simulink model "IntegrationTestSim"  (R2018b)
settings: Solver=ode45  StartTime=0.0  StopTime=600  RelTol=1e-3  EnableMultiTasking=on
values from neighbouring files (symbols this model uses):
  enableHorzMan = 1    [IntegrationTestClass.m]
  enableVertMan = 0    [IntegrationTestClass.m]
  ignorePrevAlert = 1    [IntegrationTestClass.m]
  sim_sampleTime = 0.1    [IntegrationTestClass.m]
  uasSensorSelected = 1    [IntegrationTestClass.m]
  uasSurveillance_sampleTime = 0.1    [IntegrationTestClass.m]
undefined symbols (not defined in the file or in its folder): ac1dyn_alt0_ft, ac1dyn_lat0_rad, ac1dyn_lon0_rad, daa_turnRate_dps, daa_vertRate_fpm, dh_flag, dh_ftps, dpsi_flag, dpsi_radps, uasPilot_altitudeK, uasPilot_altitudeOffset, uasPilot_altitudeTheta, uasPilot_coordDelayK, uasPilot_coordDelayMin, uasPilot_coordDelayTheta, uasPilot_desiredTurnRate_dps, uasPilot_desiredVertRate_ftpm, uasPilot_deterministicMode, uasPilot_dt_s, uasPilot_executionDelayMin, uasPilot_executionDelayMu, uasPilot_initialDelayMin, uasPilot_initialDelayMu, uasPilot_maxRelativeHdg, uasPilot_meanUpdateTimes, uasPilot_mentalFilter_climbThresh_fps, uasPilot_mentalFilter_numSamp, uasPilot_mentalFilter_turnThresh_rad, uasPilot_minUpdateTimes, uasPilot_operatorEnabled, uasPilot_probDescend, uasPilot_probFollowMinDev, uasPilot_probLeftTurn, uasPilot_probTurn, uasPilot_reducedClimbAlt_ft, uasPilot_reducedTurnAngle_deg, uasPilot_seedChoose, uasPilot_seedCoordDelay, uasPilot_seedExecutionDelay, uasPilot_seedInitialDelay, uasPilot_seedTurn, uasPilot_seedUpdate, uasPilot_seedVertical, uasPilot_triggerLevel, uasPilot_turnK, uasPilot_turnOffset, uasPilot_turnTheta
libraries: simulink x4, BasicAircraftDynamicsBlock x3, NominalTrajectory x2, FlattenAircraftEstimateBus x2, PerfectSurveillanceBlock x2, sph2cart x2, DaidalusV201Block x1, HysteresisFilterBlock x1, MofNFilterBlock x1, CommonMetricsBlock x1, SLoWCBlock x1, WellClearMetricsBlock x1
(part 3 of 3)

== system IntegrationTestSim/Surveillance Source/Subsystem/Simple Tracked Surveillance ==
  Intruder Aircraft State : Inport
  Clock : Inport  Port=2
  Intruder Aircraft State Rate : Inport  Port=3
  Rate Transition : RateTransition  OutPortSampleTime=uasLogic_sampleTime
  Rate Transition1 : RateTransition  OutPortSampleTime=uasLogic_sampleTime
  Rate Transition2 : RateTransition  OutPortSampleTime=uasLogic_sampleTime
  Simple Tracked Surveillance : SimpleTrackedSurveillanceBlock/Simple Tracked Surveillance  horizontal_position_jitter_stddev_ft=ac1_ac2_horizontal_position_jitter_stddev_ft  vertical_position_jitter_stddev_ft=ac1_ac2_vertical_position_jitter_stddev_ft  horizontal_velocity_jitter_stddev_fps=ac1_ac2_horizontal_velocity_jitter_stddev_fps  vertical_velocity_jitter_stddev_fps=ac1_ac2_vertical_velocity_jitter_stddev_fps  nVar_ft2=ac1_ac2_nVar_ft2  eVar_ft2=ac1_ac2_eVar_ft2  hVar_ft2=ac1_ac2_hVar_ft2  dnVar_ft2ps2=ac1_ac2_dnVar_ft2ps2  deVar_ft2ps2=ac1_ac2_deVar_ft2ps2  dhVar_ft2ps2=ac1_ac2_dhVar_ft2ps2  seed1=ac1_ac2_seed1  seed2=ac1_ac2_seed2  seed3=ac1_ac2_seed3  seed4=ac1_ac2_seed4  seed5=ac1_ac2_seed5  seed6=ac1_ac2_seed6  east_position_error_ft=ac1_ac2_east_position_error_ft  north_position_error_ft=ac1_ac2_north_position_error_ft  vertical_position_error_ft=ac1_ac2_vertical_position_error_ft  east_velocity_error_fps=ac1_ac2_east_velocity_error_fps  north_velocity_error_fps=ac1_ac2_north_velocity_error_fps  vertical_velocity_error_fps=ac1_ac2_vertical_velocity_error_fps  lat0_rad=ac1dyn_lat0_rad  lon0_rad=ac1dyn_lon0_rad  alt0_ft=ac1dyn_alt0_ft
  Terminator : Terminator
  Intruder AircraftEstimate : Outport
  wires:
  Intruder Aircraft State/1 -> Rate Transition/1
  Intruder Aircraft State Rate/1 -> Rate Transition2/1
  Clock/1 -> Rate Transition1/1
  Simple Tracked Surveillance/2 -> Terminator/1
  Rate Transition/1 -> Simple Tracked Surveillance/1
  Rate Transition1/1 -> Simple Tracked Surveillance/2
  Rate Transition2/1 -> Simple Tracked Surveillance/3
  Simple Tracked Surveillance/1 -> Intruder AircraftEstimate/1

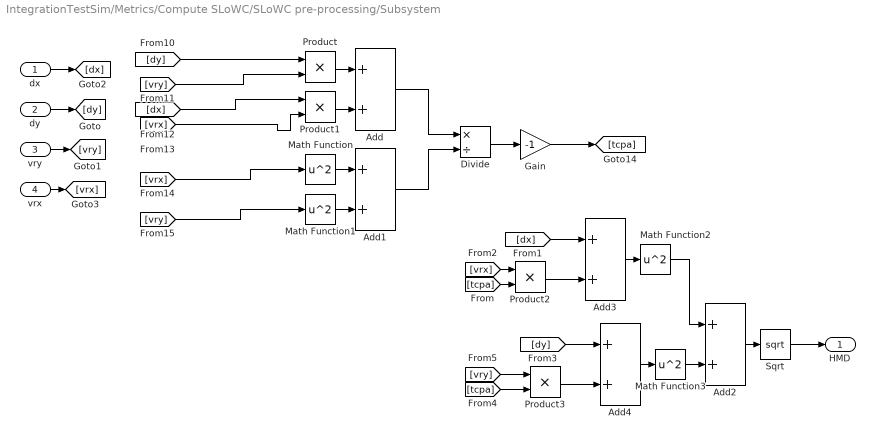
== system IntegrationTestSim/Metrics/Compute SLoWC/SLoWC pre-processing/Subsystem ==
  "dx " : Inport
  dy : Inport  Port=2
  vry : Inport  Port=3
  vrx : Inport  Port=4
  Add{,1..4} (5 alike) : Sum
  Divide : Product  Inputs=*/
  Gain : Gain  Gain=-1
  Math Function{,1..3} (4 alike) : Math  Operator=square  SaturateOnIntegerOverflow=on
  Product{,1..3} (4 alike) : Product
  Sqrt : Sqrt  SaturateOnIntegerOverflow=on
  HMD : Outport
  wires:
  Math Function1/1 -> Add1/2
  Gain/1 -> [tcpa]
  Add/1 -> Divide/1
  Math Function/1 -> Add1/1
  Product1/1 -> Add/2
  Product/1 -> Add/1
  [vrx] -> Math Function/1
  [vrx] -> Product1/2
  [dx] -> Product1/1
  Divide/1 -> Gain/1
  Add1/1 -> Divide/2
  [vry] -> Product/2
  [dy] -> Product/1
  [vry] -> Math Function1/1
  Sqrt/1 -> HMD/1
  Add2/1 -> Sqrt/1
  Math Function2/1 -> Add2/1
  Add3/1 -> Math Function2/1
  [dx] -> Add3/1
  [vrx] -> Product2/1
  Product2/1 -> Add3/2
  [tcpa] -> Product2/2
  Add4/1 -> Math Function3/1
  Math Function3/1 -> Add2/2
  Product3/1 -> Add4/2
  [dy] -> Add4/1
  [tcpa] -> Product3/2
  [vry] -> Product3/1
  "dx "/1 -> [dx]
  vrx/1 -> [vrx]
  vry/1 -> [vry]
  dy/1 -> [dy]

== system IntegrationTestSim/Metrics/Compute SLoWC/SLoWC pre-processing/Subsystem1 ==
  "int_n " : Inport
  own_n : Inport  Port=2
  int_e : Inport  Port=3
  own_e : Inport  Port=4
  Add1 : Sum
  Math Function : Math  Operator=square  SaturateOnIntegerOverflow=on
  Math Function1 : Math  Operator=square  SaturateOnIntegerOverflow=on
  Sqrt : Sqrt  SaturateOnIntegerOverflow=on
  Subtract5 : Sum  Inputs=+-
  Subtract6 : Sum  Inputs=+-
  Out1 : Outport
  wires:
  Math Function/1 -> Add1/1
  Add1/1 -> Sqrt/1
  Math Function1/1 -> Add1/2
  Subtract5/1 -> Math Function/1
  Sqrt/1 -> Out1/1
  Subtract6/1 -> Math Function1/1
  int_e/1 -> Subtract6/1
  own_n/1 -> Subtract5/2
  "int_n "/1 -> Subtract5/1
  own_e/1 -> Subtract6/2

== system IntegrationTestSim/Pilot/Format Maneuver As AircraftCommand/Horizontal Maneuver/Set Desired Turn Rate ==
  Cmd In : Inport
  Maneuver Magnitude : Inport  Port=2
  Own State : Inport  Port=3
  Bus Assignment1 : BusAssignment  AssignedSignals=dpsi_flag,dpsi_radps
  Constant : Constant  OutDataTypeStr=boolean
  Desired Heading to Turn Rate : Subsystem
  Cmd Out : Outport
  wires:
  Own State/1 -> Desired Heading to Turn Rate/2(Own State)
  Bus Assignment1/1 -> Cmd Out/1
  Cmd In/1 -> Bus Assignment1/1
  Constant/1 -> Bus Assignment1/2
  Maneuver Magnitude/1 -> Desired Heading to Turn Rate/1(Heading Cmd)
  Desired Heading to Turn Rate/1(Turn Rate) -> Bus Assignment1/3

== system IntegrationTestSim/Pilot/Format Maneuver As AircraftCommand/Vertical Maneuver/Set Desired Vertical Rate ==
  Cmd In : Inport
  Own State : Inport  Port=2
  Maneuver : Inport  Port=3
  dh_ftps : Inport  Port=4
  Bus Assignment : BusAssignment  AssignedSignals=dh_flag,dh_ftps
  Constant : Constant  OutDataTypeStr=boolean
  Constant1 : Constant  Value=enableVertMan
  Desired Altitude to Vertical Rate : Subsystem
  Multiport Switch : MultiPortSwitch  DataPortOrder=Specify indices  DataPortIndices={1 0}
  Scope : Scope
  Cmd Out : Outport
  wires:
  Bus Assignment/1 -> Cmd Out/1
  Own State/1 -> Desired Altitude to Vertical Rate/2(Own State)
  Cmd In/1 -> Bus Assignment/1
  Constant/1 -> Bus Assignment/2
  Maneuver/1 -> Desired Altitude to Vertical Rate/1(Altitude Cmd)
  dh_ftps/1 -> Multiport Switch/3
  Constant1/1 -> Multiport Switch/1
  Desired Altitude to Vertical Rate/1(Vert Rt) -> Scope/1, Multiport Switch/2
  Multiport Switch/1 -> Bus Assignment/3

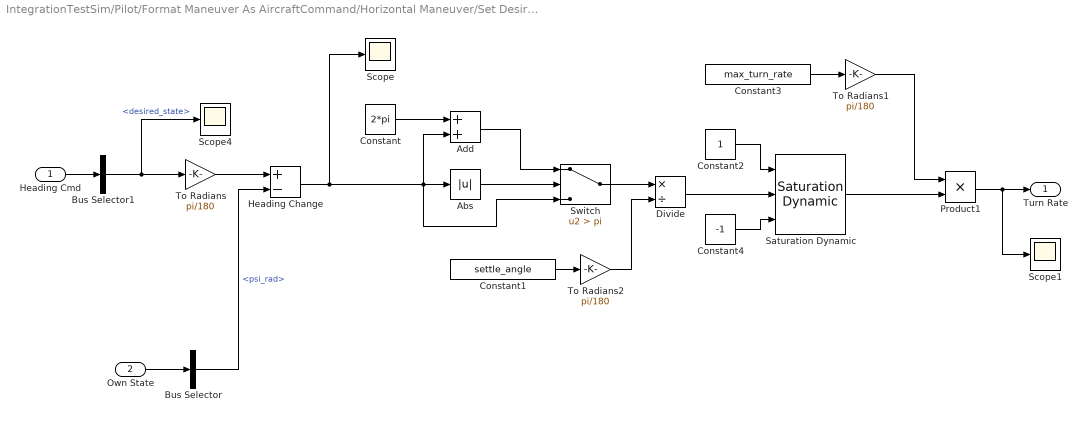
== system IntegrationTestSim/Pilot/Format Maneuver As AircraftCommand/Horizontal Maneuver/Set Desired Turn Rate/Desired Heading to Turn Rate ==
  Heading Cmd : Inport
  Own State : Inport  Port=2
  Abs : Abs
  Add : Sum
  Bus Selector : BusSelector  OutputSignals=psi_rad
  Bus Selector1 : BusSelector  OutputSignals=desired_state
  Constant : Constant  Value=2*pi
  Constant1 : Constant  Value=settle_angle
  Constant2 : Constant
  Constant3 : Constant  Value=max_turn_rate
  Constant4 : Constant  Value=-1
  Divide : Product  Inputs=*/
  Heading Change : Sum  Inputs=+-
  Product1 : Product  RndMeth=Zero
  Saturation Dynamic : simulink/Discontinuities/Saturation Dynamic  OutMin=[]  OutMax=[]  OutDataTypeStr=Inherit: Same as second input  OutDataType=fixdt(1, 16)  OutScaling=2^-10  DoSatur=off
  Scope : Scope
  Scope1 : Scope
  Scope4 : Scope
  Switch : Switch  Criteria=u2 > Threshold  Threshold=pi
  To Radians : Gain  Gain=pi/180
  To Radians1 : Gain  Gain=pi/180
  To Radians2 : Gain  Gain=pi/180
  Turn Rate : Outport
  wires:
  Constant/1 -> Add/1
  Switch/1 -> Divide/1
  Constant4/1 -> Saturation Dynamic/3
  Divide/1 -> Saturation Dynamic/2
  Abs/1 -> Switch/2
  Heading Change/1 -> Scope/1, Switch/3, Abs/1, Add/2
  Add/1 -> Switch/1
  Own State/1 -> Bus Selector/1
  Bus Selector/1 -> Heading Change/2  "<psi_rad>"
  To Radians/1 -> Heading Change/1
  Constant2/1 -> Saturation Dynamic/1
  Saturation Dynamic/1 -> Product1/2
  Constant1/1 -> To Radians2/1
  Product1/1 -> Scope1/1, Turn Rate/1
  Constant3/1 -> To Radians1/1
  To Radians1/1 -> Product1/1
  To Radians2/1 -> Divide/2
  Bus Selector1/1 -> To Radians/1, Scope4/1  "<desired_state>"
  Heading Cmd/1 -> Bus Selector1/1

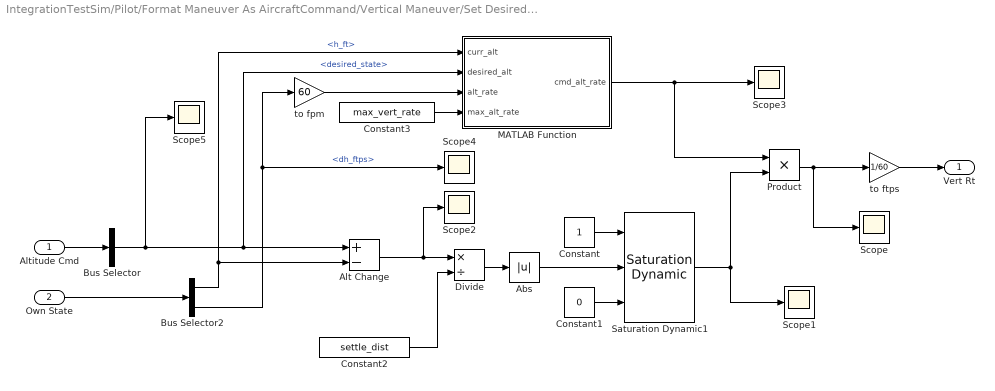
== system IntegrationTestSim/Pilot/Format Maneuver As AircraftCommand/Vertical Maneuver/Set Desired Vertical Rate/Desired Altitude to Vertical Rate ==
  Altitude Cmd : Inport
  Own State : Inport  Port=2
  Abs : Abs
  Alt Change : Sum  Inputs=+-
  Bus Selector : BusSelector  OutputSignals=desired_state
  Bus Selector2 : BusSelector  OutputSignals=h_ft,dh_ftps
  Constant : Constant
  Constant1 : Constant  Value=0
  Constant2 : Constant  Value=settle_dist
  Constant3 : Constant  Value=max_vert_rate
  Divide : Product  Inputs=*/
  MATLAB Function : MATLAB Function  TreatAsAtomicUnit=on
  Product : Product  RndMeth=Zero
  Saturation Dynamic1 : simulink/Discontinuities/Saturation Dynamic  OutMin=[]  OutMax=[]  OutDataTypeStr=Inherit: Same as second input  OutDataType=fixdt(1, 16)  OutScaling=2^-10  DoSatur=off
  Scope{,1..5} (6 alike) : Scope
  to fpm : Gain  Gain=60
  to ftps : Gain  Gain=1/60
  Vert Rt : Outport
  wires:
  Constant2/1 -> Divide/2
  Alt Change/1 -> Divide/1, Scope2/1
  Product/1 -> to ftps/1, Scope/1
  Own State/1 -> Bus Selector2/1
  Altitude Cmd/1 -> Bus Selector/1
  Bus Selector2/1 -> MATLAB Function/1(curr_alt), Alt Change/2  "<h_ft>"
  Divide/1 -> Abs/1
  Constant/1 -> Saturation Dynamic1/1
  Constant1/1 -> Saturation Dynamic1/3
  Saturation Dynamic1/1 -> Scope1/1, Product/2
  Abs/1 -> Saturation Dynamic1/2
  to ftps/1 -> Vert Rt/1
  Bus Selector/1 -> Scope5/1, MATLAB Function/2(desired_alt), Alt Change/1  "<desired_state>"
  Constant3/1 -> MATLAB Function/4(max_alt_rate)
  Bus Selector2/2 -> Scope4/1, to fpm/1  "<dh_ftps>"
  MATLAB Function/1(cmd_alt_rate) -> Scope3/1, Product/1
  to fpm/1 -> MATLAB Function/3(alt_rate)

== matlab function IntegrationTestSim/Surveillance Source/Subsystem/SC-228 Active Surveillance (Tracked)/MATLAB Function ==
  data: lat0 input double; lon0 input double; h0 input double; n_ft input double; e_ft input double size=1; u_ft input double; vn_ftps input double; ve_ftps input double; vh_ftps input double; lat_rad output double; lon_rad output double; dlat_radps output double; dlon_radps output double; alt_ft output double; dalt_ftps output double
function [lat_rad,lon_rad,dlat_radps,dlon_radps,alt_ft,dalt_ftps] = convertToLLA(lat0,lon0,h0,n_ft,e_ft,u_ft,vn_ftps,ve_ftps,vh_ftps)
%#codegen

% WGS-84 ellipsoid constants
a = 2.09256*10^7;          %Semi-major axis (meters)
f = 1.0/298.257223563;  %Flattening
ecc_sq = f*(2.0-f);        %Eccentricity^2


% Ellipsoidal "radius"
er = a./sqrt(1-ecc_sq.*sin(lat0).^2);


% ECEF coordinates
x0 = (er + h0)*cos(lat0)*cos(lon0);
y0 = (er + h0)*cos(lat0)*sin(lon0);
z0 = (er.*(1-ecc_sq) + h0)*sin(lat0);


%% Rotation Matrix
posECEF0 = [x0;y0;z0];
% Compute the local Up unit vector
vHatU = posECEF0;
vHatU(3) = vHatU(3) ./ ((1-f)^2);
vHatU = vHatU ./ norm(vHatU);

% Compute the projection onto the local Up vector
pU = vHatU * vHatU';

% Compute the projection onto the local Tangent plane
pT = eye(size(pU)) - pU;

% Compute the local North unit vector
vHatZ = [0;0;1];
vHatN = pT * vHatZ;
vHatN = vHatN ./ norm(vHatN);

% Compute the local East unit vector
vHatE = cross(vHatN,vHatU);

% Compute ENU rotation matrix
rotMatENU = zeros(3,3);
rotMatENU(:,1) = vHatE;
rotMatENU(:,2) = vHatN;
rotMatENU(:,3) = vHatU;

tPosECEF = rotMatENU*[e_ft;n_ft;u_ft] + [x0;y0;z0];


%% ECEF to LLA
% WGS-84 derived parameters
b = (1-f).*a;                       %Semi-minor axis (meters)
ecc1_sq = (a.^2 - b.^2)./(a.^2);    %First eccentricity squared
ecc2_sq = (a.^2 - b.^2)./(b.^2);    %Second eccentricity squared


% Length of position vector in equatorial plane
rho = sqrt(tPosECEF(1).^2 + tPosECEF(2).^2);

% Auxillary angle
theta = atan( (tPosECEF(3).*a)./(rho.*b) );

lon_rad = atan2(tPosECEF(2),tPosECEF(1));
lat_rad = atan( (tPosECEF(3) + ecc2_sq.*b.*(sin(theta)).^3)./(rho - ecc1_sq.*a.*(cos(theta)).^3) );

ewRadCurv = a./sqrt(1-ecc1_sq.*sin(lat_rad).^2);

alt_ft = (rho./cos(lat_rad)) - ewRadCurv;


%% Velocities - Project 1 sec into future and use to estimate
dalt_ftps = vh_ftps; % Assume about the same


tPosECEF_1sec = rotMatENU*[e_ft+ve_ftps;...
                           n_ft+vn_ftps;...
                           u_ft] + ...
                           [x0;y0;z0];

% Length of position vector in equatorial plane
rho = sqrt(tPosECEF_1sec(1).^2 + tPosECEF_1sec(2).^2);

% Auxillary angle
theta = atan( (tPosECEF_1sec(3).*a)./(rho.*b) );

lon_rad_1sec = atan2(tPosECEF_1sec(2),tPosECEF_1sec(1));
lat_rad_1sec = atan( (tPosECEF_1sec(3) + ecc2_sq.*b.*(sin(theta)).^3)./(rho - ecc1_sq.*a.*(cos(theta)).^3) );

dlat_radps = lat_rad_1sec - lat_rad;
dlon_radps = lon_rad_1sec - lon_rad;
end

== matlab function IntegrationTestSim/Pilot/Horizontal and Vertical guidance enabler/Vertical Band manipulation ==
  data: Guidance_in input; Guidance_out output
function Guidance_out = fcn(Guidance_in)

temp = Guidance_in;
temp(273) = 4;
temp(275) = 4;
temp(277) = 4;
temp(279) = 4;
temp(281) = 4;
temp(283) = 4;

Guidance_out = temp;

== matlab function IntegrationTestSim/Pilot/Horizontal and Vertical guidance enabler/Horizontal Band manipulation ==
  data: Guidance_in input; Guidance_out output
function Guidance_out = fcn(Guidance_in)

temp = Guidance_in;
temp(1:271) = 4;

Guidance_out = temp;

== matlab function IntegrationTestSim/Surveillance Source/Subsystem/SC-228 Active Surveillance (Tracked)/cyl2xyz ==
  data: x output; r input; y output; rDot input; b input; bDot input; h input; hDot input; ownPsi input; ownPsiDot input; z output; xDot output; yDot output; zDot output; J output; K output
function [x,y,z,xDot,yDot,zDot,J,K] = fcn(r,rDot,b,bDot,h,hDot,ownPsi,ownPsiDot)
%#codegen
% Convert position and velocity of intruder relative to ownship from 
% range/bearing/altitude coordinates to North-East-Down coordinates. Also
% returns Jacobian blocks J and K, where 6x6 Jacobian = [J zeros; K J]

% because of independent noise, it's possible that estimated range can be
% smaller than estimated altitude --  in that case, use a range just
% slightly larger than the altitude
if abs(r) < abs(h)
    if r==0
        r = abs(h)+1;
    else
        r = sign(r)*abs(h)+1;
    end
end

r2D = sqrt(r^2 - h^2);

x = r2D*cos(b+ownPsi);
y = r2D*sin(b+ownPsi);
z = -h;

xDot = (1/r2D)*((r*rDot - h*hDot)*cos(b + ownPsi) - r2D*sin(b + ownPsi)*(bDot + ownPsiDot));
yDot = (1/r2D)*((r*rDot - h*hDot)*sin(b + ownPsi) + r2D*cos(b + ownPsi)*(bDot + ownPsiDot));
zDot = -hDot;

% Jacobian elements (for xyz -> cyl)

J = [  x/r   y/r    z/r ;
     -y/r2D^2  x/r2D^2   0  ;
          0       0 -1 ];
      
K = zeros(3,3);
K(1,1) = xDot/r - x*rDot/r^2;
K(1,2) = yDot/r - y*rDot/r^2;
K(1,3) = zDot/r - z*rDot/r^2;
K(2,1) = (yDot*y^2 + 2*x*xDot*y - yDot*x^2)/r2D^4;
K(2,2) = (xDot*y^2 - 2*x*y*yDot - x^2*xDot)/r2D^4;

% use Schur complement for cyl -> xyz
if ~isnan(rcond(J))
  J = inv(J);
  K = -J*K*J;
else
  J = nan(3);
  K = nan(3);
end

== matlab function IntegrationTestSim/Surveillance Source/Subsystem/SC-228 Radar Model (Tracked)/MATLAB Function ==
  data: lat0 input double; lon0 input double; h0 input double; n_ft input double; e_ft input double size=1; u_ft input double; vn_ftps input double; ve_ftps input double; vh_ftps input double; lat_rad output double; lon_rad output double; dlat_radps output double; dlon_radps output double; alt_ft output double; dalt_ftps output double
function [lat_rad,lon_rad,dlat_radps,dlon_radps,alt_ft,dalt_ftps] = convertToLLA(lat0,lon0,h0,n_ft,e_ft,u_ft,vn_ftps,ve_ftps,vh_ftps)
%#codegen

% WGS-84 ellipsoid constants
a = 2.09256*10^7;          %Semi-major axis (meters)
f = 1.0/298.257223563;  %Flattening
ecc_sq = f*(2.0-f);        %Eccentricity^2


% Ellipsoidal "radius"
er = a./sqrt(1-ecc_sq.*sin(lat0).^2);


% ECEF coordinates
x0 = (er + h0)*cos(lat0)*cos(lon0);
y0 = (er + h0)*cos(lat0)*sin(lon0);
z0 = (er.*(1-ecc_sq) + h0)*sin(lat0);


%% Rotation Matrix
posECEF0 = [x0;y0;z0];
% Compute the local Up unit vector
vHatU = posECEF0;
vHatU(3) = vHatU(3) ./ ((1-f)^2);
vHatU = vHatU ./ norm(vHatU);

% Compute the projection onto the local Up vector
pU = vHatU * vHatU';

% Compute the projection onto the local Tangent plane
pT = eye(size(pU)) - pU;

% Compute the local North unit vector
vHatZ = [0;0;1];
vHatN = pT * vHatZ;
vHatN = vHatN ./ norm(vHatN);

% Compute the local East unit vector
vHatE = cross(vHatN,vHatU);

% Compute ENU rotation matrix
rotMatENU = zeros(3,3);
rotMatENU(:,1) = vHatE;
rotMatENU(:,2) = vHatN;
rotMatENU(:,3) = vHatU;

tPosECEF = rotMatENU*[e_ft;n_ft;u_ft] + [x0;y0;z0];


%% ECEF to LLA
% WGS-84 derived parameters
b = (1-f).*a;                       %Semi-minor axis (meters)
ecc1_sq = (a.^2 - b.^2)./(a.^2);    %First eccentricity squared
ecc2_sq = (a.^2 - b.^2)./(b.^2);    %Second eccentricity squared


% Length of position vector in equatorial plane
rho = sqrt(tPosECEF(1).^2 + tPosECEF(2).^2);

% Auxillary angle
theta = atan( (tPosECEF(3).*a)./(rho.*b) );

lon_rad = atan2(tPosECEF(2),tPosECEF(1));
lat_rad = atan( (tPosECEF(3) + ecc2_sq.*b.*(sin(theta)).^3)./(rho - ecc1_sq.*a.*(cos(theta)).^3) );

ewRadCurv = a./sqrt(1-ecc1_sq.*sin(lat_rad).^2);

alt_ft = (rho./cos(lat_rad)) - ewRadCurv;


%% Velocities - Project 1 sec into future and use to estimate
dalt_ftps = vh_ftps; % Assume about the same


tPosECEF_1sec = rotMatENU*[e_ft+ve_ftps;...
                           n_ft+vn_ftps;...
                           u_ft] + ...
                           [x0;y0;z0];

% Length of position vector in equatorial plane
rho = sqrt(tPosECEF_1sec(1).^2 + tPosECEF_1sec(2).^2);

% Auxillary angle
theta = atan( (tPosECEF_1sec(3).*a)./(rho.*b) );

lon_rad_1sec = atan2(tPosECEF_1sec(2),tPosECEF_1sec(1));
lat_rad_1sec = atan( (tPosECEF_1sec(3) + ecc2_sq.*b.*(sin(theta)).^3)./(rho - ecc1_sq.*a.*(cos(theta)).^3) );

dlat_radps = lat_rad_1sec - lat_rad;
dlon_radps = lon_rad_1sec - lon_rad;
end

== matlab function IntegrationTestSim/Surveillance Source/Subsystem/SC-228 Radar Model/NED2FRD ==
  data: psi_rad input; T output; theta input; phi input
function T = Transform_NED2FRD(psi_rad,theta,phi)
%#codegen

yaw = [ cos(psi_rad) sin(psi_rad) 0;
       -sin(psi_rad) cos(psi_rad) 0;
               0        0 1 ];
           
pitch = [ cos(theta) 0 -sin(theta);
                   0 1           0;
          sin(theta) 0  cos(theta) ];
      
roll = [ 1         0        0;
         0  cos(phi) sin(phi);
         0 -sin(phi) cos(phi) ];
     
T = roll*pitch*yaw;     % transformation FROM geographic coord TO body coord

== matlab function IntegrationTestSim/Surveillance Source/Subsystem/SC-228 Radar Model/MATLAB Function ==
  data: lat0 input double; lon0 input double; h0 input double; n_ft input double; e_ft input double size=1; u_ft input double; vn_ftps input double; ve_ftps input double; vh_ftps input double; lat_rad output double; lon_rad output double; dlat_radps output double; dlon_radps output double; alt_ft output double; dalt_ftps output double
function [lat_rad,lon_rad,dlat_radps,dlon_radps,alt_ft,dalt_ftps] = convertToLLA(lat0,lon0,h0,n_ft,e_ft,u_ft,vn_ftps,ve_ftps,vh_ftps)
%#codegen

% WGS-84 ellipsoid constants
a = 2.09256*10^7;          %Semi-major axis (meters)
f = 1.0/298.257223563;  %Flattening
ecc_sq = f*(2.0-f);        %Eccentricity^2


% Ellipsoidal "radius"
er = a./sqrt(1-ecc_sq.*sin(lat0).^2);


% ECEF coordinates
x0 = (er + h0)*cos(lat0)*cos(lon0);
y0 = (er + h0)*cos(lat0)*sin(lon0);
z0 = (er.*(1-ecc_sq) + h0)*sin(lat0);


%% Rotation Matrix
posECEF0 = [x0;y0;z0];
% Compute the local Up unit vector
vHatU = posECEF0;
vHatU(3) = vHatU(3) ./ ((1-f)^2);
vHatU = vHatU ./ norm(vHatU);

% Compute the projection onto the local Up vector
pU = vHatU * vHatU';

% Compute the projection onto the local Tangent plane
pT = eye(size(pU)) - pU;

% Compute the local North unit vector
vHatZ = [0;0;1];
vHatN = pT * vHatZ;
vHatN = vHatN ./ norm(vHatN);

% Compute the local East unit vector
vHatE = cross(vHatN,vHatU);

% Compute ENU rotation matrix
rotMatENU = zeros(3,3);
rotMatENU(:,1) = vHatE;
rotMatENU(:,2) = vHatN;
rotMatENU(:,3) = vHatU;

tPosECEF = rotMatENU*[e_ft;n_ft;u_ft] + [x0;y0;z0];


%% ECEF to LLA
% WGS-84 derived parameters
b = (1-f).*a;                       %Semi-minor axis (meters)
ecc1_sq = (a.^2 - b.^2)./(a.^2);    %First eccentricity squared
ecc2_sq = (a.^2 - b.^2)./(b.^2);    %Second eccentricity squared


% Length of position vector in equatorial plane
rho = sqrt(tPosECEF(1).^2 + tPosECEF(2).^2);

% Auxillary angle
theta = atan( (tPosECEF(3).*a)./(rho.*b) );

lon_rad = atan2(tPosECEF(2),tPosECEF(1));
lat_rad = atan( (tPosECEF(3) + ecc2_sq.*b.*(sin(theta)).^3)./(rho - ecc1_sq.*a.*(cos(theta)).^3) );

ewRadCurv = a./sqrt(1-ecc1_sq.*sin(lat_rad).^2);

alt_ft = (rho./cos(lat_rad)) - ewRadCurv;


%% Velocities - Project 1 sec into future and use to estimate
dalt_ftps = vh_ftps; % Assume about the same


tPosECEF_1sec = rotMatENU*[e_ft+ve_ftps;...
                           n_ft+vn_ftps;...
                           u_ft] + ...
                           [x0;y0;z0];

% Length of position vector in equatorial plane
rho = sqrt(tPosECEF_1sec(1).^2 + tPosECEF_1sec(2).^2);

% Auxillary angle
theta = atan( (tPosECEF_1sec(3).*a)./(rho.*b) );

lon_rad_1sec = atan2(tPosECEF_1sec(2),tPosECEF_1sec(1));
lat_rad_1sec = atan( (tPosECEF_1sec(3) + ecc2_sq.*b.*(sin(theta)).^3)./(rho - ecc1_sq.*a.*(cos(theta)).^3) );

dlat_radps = lat_rad_1sec - lat_rad;
dlon_radps = lon_rad_1sec - lon_rad;
end

== matlab function IntegrationTestSim/Pilot/Format Maneuver As AircraftCommand/Vertical Maneuver/Set Desired Vertical Rate/Desired Altitude to Vertical Rate/MATLAB Function ==
  data: curr_alt input; cmd_alt_rate output; desired_alt input; alt_rate input; max_alt_rate input
function cmd_alt_rate = fcn(curr_alt, desired_alt, alt_rate, max_alt_rate)
%#codegen

if desired_alt >= curr_alt
  cmd_alt_rate = max_alt_rate;
else
  cmd_alt_rate = -max_alt_rate;
end

% override specified vertical rate for maneuvers if already climbing or
% descending in direction of desired altitude

% currently climbing
% if alt_rate > 0
%   
%   if desired_alt > curr_alt
%     cmd_alt_rate = alt_rate;
%   end
%   
% % currently descending
% elseif alt_rate < 0
%   
%   if desired_alt < curr_alt
%     cmd_alt_rate = alt_rate;
%   end
%   
% end

== matlab function IntegrationTestSim/Metrics/Compute SLoWC/SLoWC pre-processing/Calculate Horizontal Proximity ==
  data: ownV input; N input; horzProx output; E input; h input; Ni input; Ei input; hi input; intV input; DMOD input; tauMod input
function horzProx = getHorzProx(ownV,N,E,h,Ni,Ei,hi,intV, DMOD, tauMod) 
% This block computes horizontal proximity (S_i in the Bihrle slide 3)

%Ri = [Ni-N; Ei-E; -(hi-h)];
Ri = [Ni-N; Ei-E; 0];

rangeRate = 0;

if(~isempty(Ri) && ~isempty(ownV) && ~isempty(intV))
    relVel = intV - ownV;
    rangeRate = dot(Ri/norm(Ri), relVel);
end

horzProx = max(DMOD, 0.5* (sqrt((rangeRate*tauMod)^2 + 4*DMOD^2) - rangeRate*tauMod) );

== matlab function IntegrationTestSim/Surveillance Source/Subsystem/SC-228 Active Surveillance/cyl2xyz ==
  data: x output; r input; y output; rDot input; b input; bDot input; h input; hDot input; ownPsi input; ownPsiDot input; z output; xDot output; yDot output; zDot output; J output; K output
function [x,y,z,xDot,yDot,zDot,J,K] = fcn(r,rDot,b,bDot,h,hDot,ownPsi,ownPsiDot)
%#codegen
% Convert position and velocity of intruder relative to ownship from 
% range/bearing/altitude coordinates to North-East-Down coordinates. Also
% returns Jacobian blocks J and K, where 6x6 Jacobian = [J zeros; K J]

% because of independent noise, it's possible that estimated range can be
% smaller than estimated altitude --  in that case, use a range just
% slightly larger than the altitude
if abs(r) < abs(h)
    if r==0
        r = abs(h)+1;
    else
        r = sign(r)*abs(h)+1;
    end
end

r2D = sqrt(r^2 - h^2);

x = r2D*cos(b+ownPsi);
y = r2D*sin(b+ownPsi);
z = -h;

xDot = (1/r2D)*((r*rDot - h*hDot)*cos(b + ownPsi) - r2D*sin(b + ownPsi)*(bDot + ownPsiDot));
yDot = (1/r2D)*((r*rDot - h*hDot)*sin(b + ownPsi) + r2D*cos(b + ownPsi)*(bDot + ownPsiDot));
zDot = -hDot;

% Jacobian elements (for xyz -> cyl)

J = [  x/r   y/r    z/r ;
     -y/r2D^2  x/r2D^2   0  ;
          0       0 -1 ];
      
K = zeros(3,3);
K(1,1) = xDot/r - x*rDot/r^2;
K(1,2) = yDot/r - y*rDot/r^2;
K(1,3) = zDot/r - z*rDot/r^2;
K(2,1) = (yDot*y^2 + 2*x*xDot*y - yDot*x^2)/r2D^4;
K(2,2) = (xDot*y^2 - 2*x*y*yDot - x^2*xDot)/r2D^4;

% use Schur complement for cyl -> xyz
if ~isnan(rcond(J))
  J = inv(J);
  K = -J*K*J;
else
  J = nan(3);
  K = nan(3);
end

== matlab function IntegrationTestSim/Surveillance Source/Subsystem/SC-228 Active Surveillance/MATLAB Function ==
  data: lat0 input double; lon0 input double; h0 input double; n_ft input double; e_ft input double size=1; u_ft input double; vn_ftps input double; ve_ftps input double; vh_ftps input double; lat_rad output double; lon_rad output double; dlat_radps output double; dlon_radps output double; alt_ft output double; dalt_ftps output double
function [lat_rad,lon_rad,dlat_radps,dlon_radps,alt_ft,dalt_ftps] = convertToLLA(lat0,lon0,h0,n_ft,e_ft,u_ft,vn_ftps,ve_ftps,vh_ftps)
%#codegen

% WGS-84 ellipsoid constants
a = 2.09256*10^7;          %Semi-major axis (meters)
f = 1.0/298.257223563;  %Flattening
ecc_sq = f*(2.0-f);        %Eccentricity^2


% Ellipsoidal "radius"
er = a./sqrt(1-ecc_sq.*sin(lat0).^2);


% ECEF coordinates
x0 = (er + h0)*cos(lat0)*cos(lon0);
y0 = (er + h0)*cos(lat0)*sin(lon0);
z0 = (er.*(1-ecc_sq) + h0)*sin(lat0);


%% Rotation Matrix
posECEF0 = [x0;y0;z0];
% Compute the local Up unit vector
vHatU = posECEF0;
vHatU(3) = vHatU(3) ./ ((1-f)^2);
vHatU = vHatU ./ norm(vHatU);

% Compute the projection onto the local Up vector
pU = vHatU * vHatU';

% Compute the projection onto the local Tangent plane
pT = eye(size(pU)) - pU;

% Compute the local North unit vector
vHatZ = [0;0;1];
vHatN = pT * vHatZ;
vHatN = vHatN ./ norm(vHatN);

% Compute the local East unit vector
vHatE = cross(vHatN,vHatU);

% Compute ENU rotation matrix
rotMatENU = zeros(3,3);
rotMatENU(:,1) = vHatE;
rotMatENU(:,2) = vHatN;
rotMatENU(:,3) = vHatU;

tPosECEF = rotMatENU*[e_ft;n_ft;u_ft] + [x0;y0;z0];


%% ECEF to LLA
% WGS-84 derived parameters
b = (1-f).*a;                       %Semi-minor axis (meters)
ecc1_sq = (a.^2 - b.^2)./(a.^2);    %First eccentricity squared
ecc2_sq = (a.^2 - b.^2)./(b.^2);    %Second eccentricity squared


% Length of position vector in equatorial plane
rho = sqrt(tPosECEF(1).^2 + tPosECEF(2).^2);

% Auxillary angle
theta = atan( (tPosECEF(3).*a)./(rho.*b) );

lon_rad = atan2(tPosECEF(2),tPosECEF(1));
lat_rad = atan( (tPosECEF(3) + ecc2_sq.*b.*(sin(theta)).^3)./(rho - ecc1_sq.*a.*(cos(theta)).^3) );

ewRadCurv = a./sqrt(1-ecc1_sq.*sin(lat_rad).^2);

alt_ft = (rho./cos(lat_rad)) - ewRadCurv;


%% Velocities - Project 1 sec into future and use to estimate
dalt_ftps = vh_ftps; % Assume about the same


tPosECEF_1sec = rotMatENU*[e_ft+ve_ftps;...
                           n_ft+vn_ftps;...
                           u_ft] + ...
                           [x0;y0;z0];

% Length of position vector in equatorial plane
rho = sqrt(tPosECEF_1sec(1).^2 + tPosECEF_1sec(2).^2);

% Auxillary angle
theta = atan( (tPosECEF_1sec(3).*a)./(rho.*b) );

lon_rad_1sec = atan2(tPosECEF_1sec(2),tPosECEF_1sec(1));
lat_rad_1sec = atan( (tPosECEF_1sec(3) + ecc2_sq.*b.*(sin(theta)).^3)./(rho - ecc1_sq.*a.*(cos(theta)).^3) );

dlat_radps = lat_rad_1sec - lat_rad;
dlon_radps = lon_rad_1sec - lon_rad;
end

== matlab function IntegrationTestSim/Surveillance Source/Subsystem/SC-228 Radar Model (Tracked)/NED2FRD ==
  data: psi_rad input; T output; theta input; phi input
function T = Transform_NED2FRD(psi_rad,theta,phi)
%#codegen

yaw = [ cos(psi_rad) sin(psi_rad) 0;
       -sin(psi_rad) cos(psi_rad) 0;
               0        0 1 ];
           
pitch = [ cos(theta) 0 -sin(theta);
                   0 1           0;
          sin(theta) 0  cos(theta) ];
      
roll = [ 1         0        0;
         0  cos(phi) sin(phi);
         0 -sin(phi) cos(phi) ];
     
T = roll*pitch*yaw;     % transformation FROM geographic coord TO body coord
